simulink model "stateflow_ROS"  (R2020a)
settings: Solver=FixedStepAuto  StartTime=0.0  StopTime=inf  RelTol=1e-3
undefined symbols (not defined in the file): Angular, Linear
libraries: robotlib x3
settings Model: Creator=pozdr  LastModifiedBy=pozdr
settings OptimizationCC: EnhancedBackFolding=on  PassReuseOutputArgsAs=Individual arguments  ZeroExternalMemoryAtStartup=off  ZeroInternalMemoryAtStartup=off  MaxStackSize=64  OptimizeBlockOrder=speed  DifferentSizesBufferReuse=on  OptimizationCustomize=off  EfficientTunableParamExpr=on
settings DebuggingCC: ParameterTunabilityLossMsg=error
settings HardwareCC: ProdBitPerPointer=32  ProdBitPerSizeT=32  ProdBitPerPtrDiffT=32  ProdLargestAtomicFloat=None  ProdIntDivRoundTo=Undefined  ProdEndianess=Unspecified  ProdWordSize=32  ProdHWDeviceType=Generic->Unspecified (assume 32-bit Generic)  UseEmbeddedCoderFeatures=off
settings SFSimCC: MATLABDynamicMemAlloc=off
settings RTWCC: SystemTargetFile=ert.tlc  HardwareBoard=Robot Operating System (ROS)  TemplateMakefile=ert_default_tmf  Toolchain=Catkin  TargetLang=C++
settings CodeAppCC: ForceParamTrailComments=on  IgnoreCustomStorageClasses=off  OperatorAnnotations=on  SimulinkDataObjDesc=on  SFDataObjDesc=on  InsertBlockDesc=on
settings ERTTargetCC: SupportNonInlinedSFcns=on

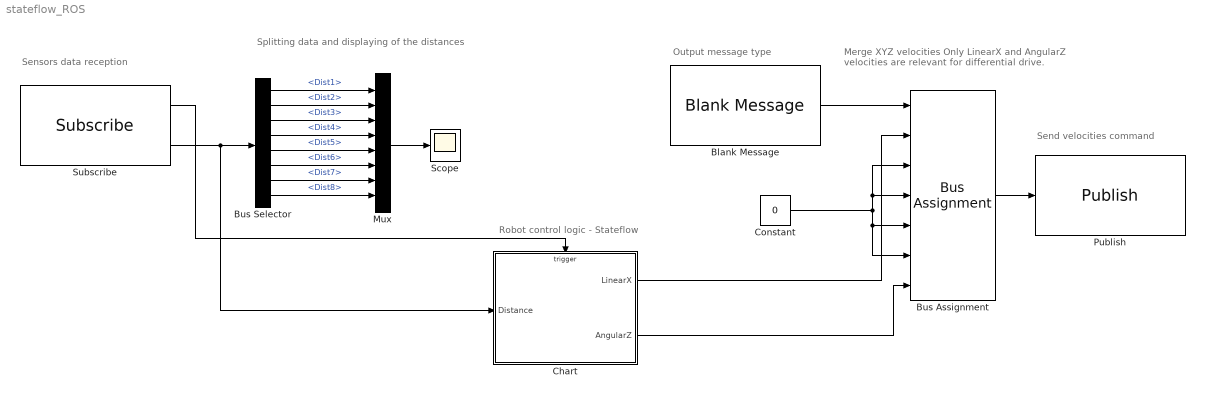
== system stateflow_ROS ==
  note: Splitting data and displaying of the distances
  note: Merge XYZ velocities
      | Only LinearX and AngularZ velocities are relevant for
      | differential drive.
  note: Send velocities command
  note: Output message type
  note: Robot control logic - Stateflow
  note: Sensors data reception
  Blank Message : robotlib/Blank Message  messageClass=Message  entityType=geometry_msgs/Twist  messageType=geometry_msgs/Twist  SampleTime=inf
  Bus Assignment : BusAssignment  AssignedSignals=Linear.X,Linear.Y,Linear.Z,Angular.X,Angular.Y,Angular.Z
  Bus Selector : BusSelector  OutputSignals=Dist1,Dist2,Dist3,Dist4,Dist5,Dist6,Dist7,Dist8
  Chart : Stateflow chart  TreatAsAtomicUnit=on
  Constant : Constant  Value=0
  Mux : Mux  Inputs=8
  Publish : robotlib/Publish  topicSource=Select from ROS network  topic=/cmd_vel  messageType=geometry_msgs/Twist  messageQueueLength=1
  Scope : Scope
  Subscribe : robotlib/Subscribe  topicSource=Select from ROS network  topic=/sensors  messageType=create_control/create_sensors  sampleTime=-1  messageQueueLength=1
  wires:
  Blank Message/1 -> Bus Assignment/1
  Bus Assignment/1 -> Publish/1
  Constant/1 -> Bus Assignment/3, Bus Assignment/4, Bus Assignment/6, Bus Assignment/5
  Subscribe/2 -> Chart/1(Distance), Bus Selector/1
  Bus Selector/2 -> Mux/2  "<Dist2>"
  Bus Selector/1 -> Mux/1  "<Dist1>"
  Bus Selector/3 -> Mux/3  "<Dist3>"
  Bus Selector/4 -> Mux/4  "<Dist4>"
  Bus Selector/5 -> Mux/5  "<Dist5>"
  Bus Selector/6 -> Mux/6  "<Dist6>"
  Bus Selector/7 -> Mux/7  "<Dist7>"
  Bus Selector/8 -> Mux/8  "<Dist8>"
  Mux/1 -> Scope/1
  Subscribe/1 -> Chart/Trigger
  Chart/1(LinearX) -> Bus Assignment/2
  Chart/2(AngularZ) -> Bus Assignment/7

== stateflow chart stateflow_ROS/Chart ==
  settings: executeAtInitialization=1
  state TurnRight
    en:LinearX = 0
    en:AngularZ = 0.1
  state Straight
    en:LinearX = 0.1
    en:AngularZ = 0
  state TurnLeft
    en:LinearX = 0
    en:AngularZ = -0.1
  (default) -> Straight
  Straight -> TurnRight [order 2] : [Distance.Dist3 < 0.5]
  Straight -> TurnLeft [order 1] : [Distance.Dist2 < 0.5]
  TurnRight -> Straight : [Distance.Dist3 > 0.7]
  TurnLeft -> Straight : [Distance.Dist2 > 0.7]
  data: Distance input; LinearX output =0; AngularZ output =0
  events: CLOCK input RISING_EDGE_EVENT
